simulink model "es2"  (R2022b)
settings: Solver=VariableStepAuto  StartTime=0.0  StopTime=10.0  RelTol=1e-3
undefined symbols (not defined in the file): A0, B0, C0, D0, den, DiscIntNeverNeededParam, K, Ki, Nu, num, Nx, sysD, T
settings Model: Creator=emanuelevitetta  LastModifiedBy=emanuelevitetta

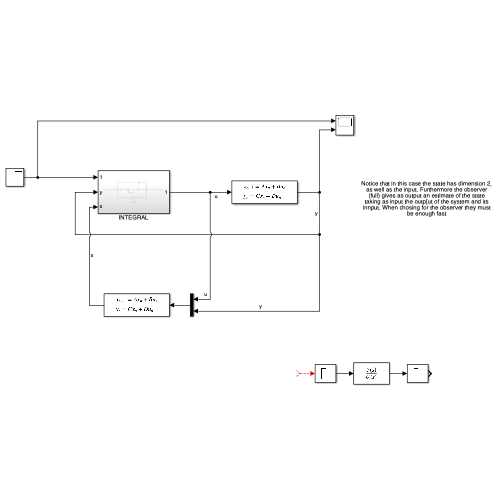
[thumbnail: Simulink's stored preview of the top-level diagram]
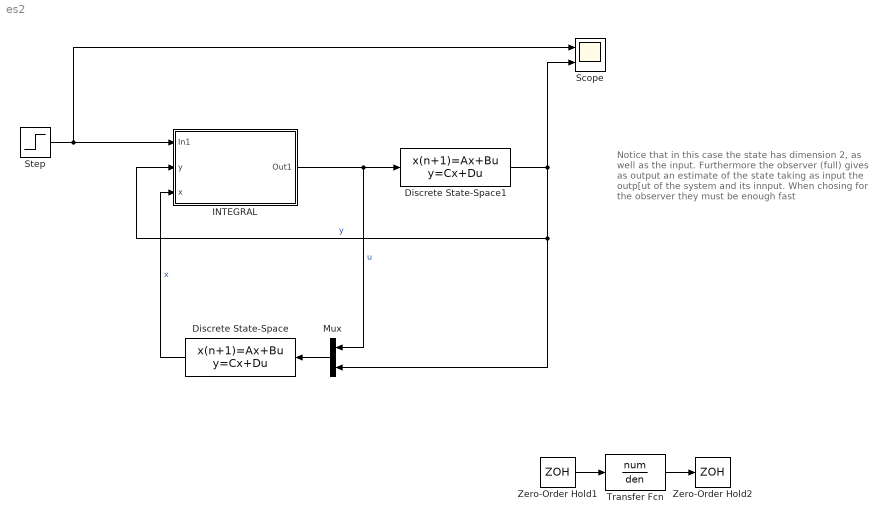
== system es2 ==
  note: Notice that in this case the state has dimension 2, as well as the input. Furthermore the observer (full) gives as output an estimate of the state taking as input the outp[ut of the system and its innput. When chosing for the observer they must be enough fast
  Discrete State-Space : DiscreteStateSpace  A=A0  B=B0  C=C0  D=D0  SampleTime=T
  Discrete State-Space1 : DiscreteStateSpace  A=sysD.A  B=sysD.B  C=sysD.C  D=sysD.D  SampleTime=-1
  INTEGRAL : Subsystem
  Mux : Mux  Inputs=2
  Scope : Scope  NumInputPorts=2
  Step : Step  After=10  SampleTime=T
  Transfer Fcn : TransferFcn  Numerator=num  Denominator=den
  Zero-Order Hold1 : ZeroOrderHold  SampleTime=T
  Zero-Order Hold2 : ZeroOrderHold  SampleTime=T
  wires:
  Discrete State-Space/1 -> INTEGRAL/3(x)  "x"
  Discrete State-Space1/1 -> Mux/2, INTEGRAL/2(y), Scope/2  "y"
  Mux/1 -> Discrete State-Space/1
  Step/1 -> INTEGRAL/1(In1), Scope/1
  INTEGRAL/1(Out1) -> Discrete State-Space1/1, Mux/1  "u"
  ? -> Zero-Order Hold1/1
  Transfer Fcn/1 -> Zero-Order Hold2/1
  Zero-Order Hold1/1 -> Transfer Fcn/1

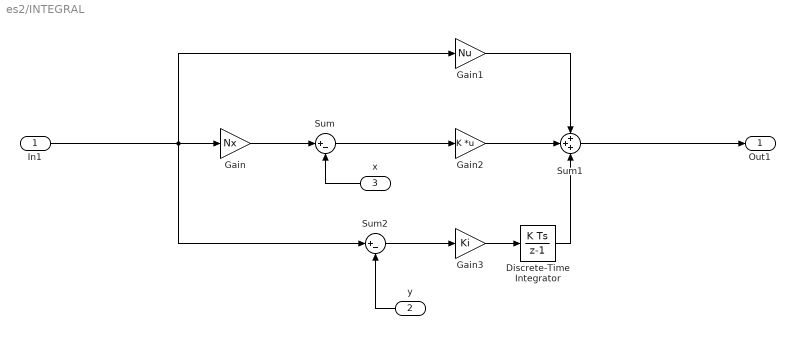
== system es2/INTEGRAL ==
  In1 : Inport
  y : Inport  Port=2
  x : Inport  Port=3
  Discrete-Time Integrator : DiscreteIntegrator  SampleTime=T  ICPrevOutput=DiscIntNeverNeededParam  ICPrevScaledInput=DiscIntNeverNeededParam
  Gain : Gain  Gain=Nx
  Gain1 : Gain  Gain=Nu
  Gain2 : Gain  Gain=K  Multiplication=Matrix(K*u)
  Gain3 : Gain  Gain=Ki
  Sum : Sum  Inputs=|+-
  Sum1 : Sum  Inputs=+++
  Sum2 : Sum  Inputs=|+-
  Out1 : Outport
  wires:
  Gain/1 -> Sum/1
  Sum/1 -> Gain2/1
  Gain2/1 -> Sum1/2
  Gain1/1 -> Sum1/1
  In1/1 -> Sum2/1, Gain1/1, Gain/1
  Sum1/1 -> Out1/1
  Discrete-Time Integrator/1 -> Sum1/3
  Gain3/1 -> Discrete-Time Integrator/1
  Sum2/1 -> Gain3/1
  y/1 -> Sum2/2
  x/1 -> Sum/2
